simulink model "rtwdemo_PCGEvalHarness"  (Simulink 7.6)
settings: Solver=FixedStepDiscrete  StartTime=0.0  StopTime=2  FixedStep=.001  RelTol=1e-3
PostLoadFcn:
  | % Load the Data
  | RTWDemos.pcgd_TestHarnessData;
StopFcn:
  | % Run the plotting script
  | if (exist('logsout','var'))
  |     RTWDemos.pcgd_plotHarnessData(logsout);
  | end
undefined symbols (not defined in the file or in its folder): A1, A2, B0, B1, B2, sigbuilder_block
libraries: simulink x1
settings Model: Creator=The MathWorks Inc.  ExtModeAutoUpdateStatusClock=off
settings DataIOCC: SaveOutput=off  SaveTime=off
settings OptimizationCC: InitFltsAndDblsToZero=on  OptimizeModelRefInitCode=on  LifeSpan=1
settings DebuggingCC: SignalResolutionControl=TryResolveAllWithWarning  StrictBusMsg=Warning
settings ModelReferenceCC: ModelReferenceNumInstancesAllowed=Single
settings RTWCC: SystemTargetFile=ert.tlc  GenCodeOnly=on  MakeCommand="make_rtw USER_INCLUDES=\"-I$matlabroot$/toolbox\\rtw\\rtwdemos\\EmbeddedCoderOverview\\stage_4_files\""  TemplateMakefile=ert_default_tmf  Description=Real-Time Workshop Embedded Coder (no auto configuration)  ProcessScript=ert_make_rtw_hook  CustomSource=SimpleTable.c
settings RTWCC: CustomInclude=|
  | $matlabroot$\toolbox\rtw\rtwdemos\EmbeddedCoderOverview\
  | $matlabroot$\toolbox\rtw\rtwdemos\EmbeddedCoderOverview\stage_4_files
settings CodeAppCC: IgnoreCustomStorageClasses=off
settings ERTTargetCC: TargetFcnLib=ansi_tfl_tmw_new.mat  MultiwordLength=2048  GenerateSampleERTMain=on  InlinedParameterPlacement=NonHierarchical  ERTCustomFileTemplate=example_file_process.tlc  ConvertIfToSwitch=off

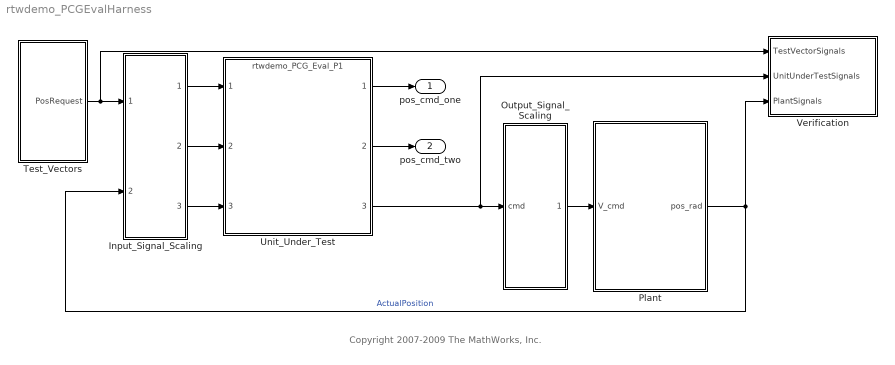
== system rtwdemo_PCGEvalHarness ==
  note: Copyright 2007-2009 The MathWorks, Inc.
  Input_Signal_Scaling : Subsystem
      mask Display:
      | disp(' ')
      | port_label('output',1,'pos_rqst');
      | port_label('output',2,'fbk_1');
      | port_label('output',3,'fbk_2');
  Output_Signal_Scaling : Subsystem
      mask Display:
      | disp(' ')
      | port_label('output',1,'pos_cmd')
  Plant : Subsystem
      mask Display: disp(' ')
  Test_Vectors : Subsystem
  Unit_Under_Test : ModelReference  ModelNameDialog=rtwdemo_PCG_Eval_P1  SimulationMode=Normal  ModelReferenceVersion=1.169  CopyOfModelName=rtwdemo_PCG_Eval_P1
  Verification : Subsystem
  pos_cmd_one : Outport
  pos_cmd_two : Outport  Port=2
  wires:
  Unit_Under_Test/3 -> Output_Signal_Scaling/1(cmd), Verification/2(UnitUnderTestSignals)
  Test_Vectors/1(PosRequest) -> Input_Signal_Scaling/1(sys_in), Verification/1(TestVectorSignals)
  Input_Signal_Scaling/1(pos_rqst) -> Unit_Under_Test/1
  Input_Signal_Scaling/2(fbk_1_out) -> Unit_Under_Test/2
  Input_Signal_Scaling/3(fbk_2_out) -> Unit_Under_Test/3
  Unit_Under_Test/1 -> pos_cmd_one/1
  Unit_Under_Test/2 -> pos_cmd_two/1
  Plant/1(pos_rad) -> Input_Signal_Scaling/2(pos_fbk), Verification/3(PlantSignals)  "ActualPosition"
  Output_Signal_Scaling/1(pos_cmd_act) -> Plant/1(V_cmd)

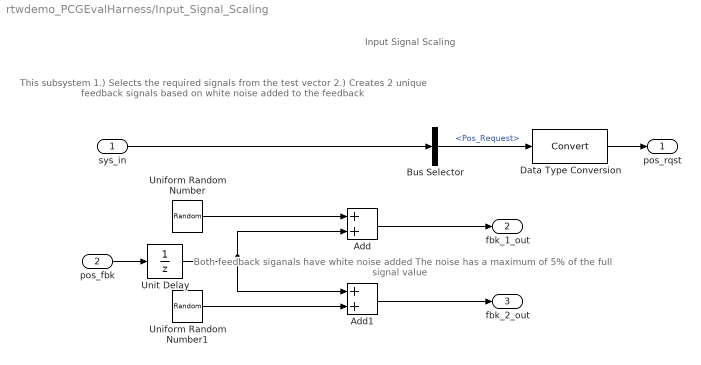
== system rtwdemo_PCGEvalHarness/Input_Signal_Scaling ==
  note: Input Signal Scaling
  note: This subsystem
      | 1.) Selects the required signals from the test vector
      | 2.) Creates 2 unique feedback signals based on white noise added to the feedback
  note: Both feedback siganals have white noise added
      | The noise has a maximum of 5% of the full signal value
  sys_in : Inport
  pos_fbk : Inport  Port=2
  Add : Sum
  Add1 : Sum
  Bus Selector : BusSelector  OutputSignals=Pos_Request
  Data Type Conversion : DataTypeConversion  SampleTime=[0.001, 0]
  Uniform Random Number : UniformRandomNumber  Minimum=-.025  Maximum=.025  SampleTime=.001
  Uniform Random Number1 : UniformRandomNumber  Minimum=-.025  Maximum=.025  Seed=10  SampleTime=.001
  Unit Delay : UnitDelay  SampleTime=-1
  pos_rqst : Outport
  fbk_1_out : Outport  Port=2
  fbk_2_out : Outport  Port=3
  wires:
  sys_in/1 -> Bus Selector/1
  Bus Selector/1 -> Data Type Conversion/1  "<Pos_Request>"
  Add/1 -> fbk_1_out/1
  Add1/1 -> fbk_2_out/1
  pos_fbk/1 -> Unit Delay/1
  Uniform Random Number/1 -> Add/1
  Uniform Random Number1/1 -> Add1/2
  Data Type Conversion/1 -> pos_rqst/1
  Unit Delay/1 -> Add/2, Add1/1

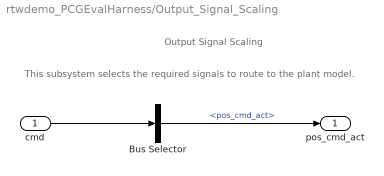
== system rtwdemo_PCGEvalHarness/Output_Signal_Scaling ==
  note: Output Signal Scaling
  note: This subsystem selects the required signals to route to the plant model.
  cmd : Inport
  Bus Selector : BusSelector  OutputSignals=pos_cmd_act
  pos_cmd_act : Outport
  wires:
  Bus Selector/1 -> pos_cmd_act/1  "<pos_cmd_act>"
  cmd/1 -> Bus Selector/1

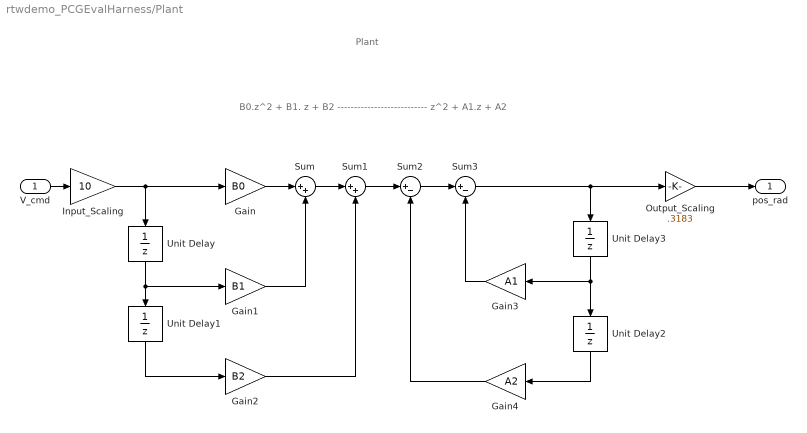
== system rtwdemo_PCGEvalHarness/Plant ==
  note: B0.z^2 + B1. z + B2
      | ---------------------------
      |    z^2 + A1.z + A2
  note: Plant
  V_cmd : Inport
  Gain : Gain  Gain=B0
  Gain1 : Gain  Gain=B1
  Gain2 : Gain  Gain=B2
  Gain3 : Gain  Gain=A1
  Gain4 : Gain  Gain=A2
  Input_Scaling : Gain  Gain=10
  Output_Scaling : Gain  Gain=.3183
  Sum : Sum  Inputs=|++
  Sum1 : Sum  Inputs=|++
  Sum2 : Sum  Inputs=|+-
  Sum3 : Sum  Inputs=|+-
  Unit Delay{,1..3} (4 alike) : UnitDelay  SampleTime=-1
  pos_rad : Outport
  wires:
  Sum2/1 -> Sum3/1
  Sum1/1 -> Sum2/1
  Gain4/1 -> Sum2/2
  Unit Delay2/1 -> Gain4/1
  Gain3/1 -> Sum3/2
  Unit Delay3/1 -> Unit Delay2/1, Gain3/1
  Sum3/1 -> Unit Delay3/1, Output_Scaling/1
  Gain2/1 -> Sum1/2
  Sum/1 -> Sum1/1
  Gain1/1 -> Sum/2
  Gain/1 -> Sum/1
  Unit Delay1/1 -> Gain2/1
  Unit Delay/1 -> Unit Delay1/1, Gain1/1
  V_cmd/1 -> Input_Scaling/1
  Output_Scaling/1 -> pos_rad/1
  Input_Scaling/1 -> Unit Delay/1, Gain/1

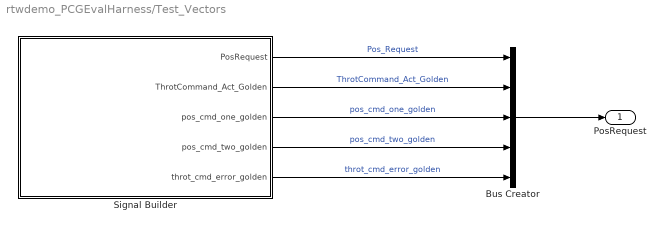
== system rtwdemo_PCGEvalHarness/Test_Vectors ==
  Bus Creator : BusCreator  Inputs=5
  Signal Builder : Subsystem  Tag=STV Subsys  LoadFcn=sigbuilder_block('load');  StartFcn=sigbuilder_block('start');  StopFcn=sigbuilder_block('stop');  ClipboardFcn=sigbuilder_block('clipboard');  mask(Sigbuilder block){}
      mask help: Sigbuilder GUI
      mask init:
      | if ~strcmp(get_param(bdroot(gcbh),'SimulationStatus'),'stopped') tuvar = sigbuilder_block('maskInit'); end
      settings: CopyFcn=sigbuilder_block('copy');  DeleteFcn=sigbuilder_block('delete');  ModelCloseFcn=sigbuilder_block('modelClose');  PreSaveFcn=sigbuilder_block('preSave');  NameChangeFcn=sigbuilder_block('namechange');  OpenFcn=sigbuilder_block('open',[0 25.5 1248 819 ]);  CloseFcn=sigbuilder_block('close');
      mask Display: plot(0,0,100,100,[10,10,40,40,10],[80,20,20,80,80],[40,10],[50,50], [40,27,10],[65,72,56],[40,25,25,10],[28,28,43,43]);
  PosRequest : Outport
  wires:
  Bus Creator/1 -> PosRequest/1
  Signal Builder/1(PosRequest) -> Bus Creator/1  "Pos_Request"
  Signal Builder/2(ThrotCommand_Act_Golden) -> Bus Creator/2  "ThrotCommand_Act_Golden"
  Signal Builder/3(pos_cmd_one_golden) -> Bus Creator/3  "pos_cmd_one_golden"
  Signal Builder/4(pos_cmd_two_golden) -> Bus Creator/4  "pos_cmd_two_golden"
  Signal Builder/5(throt_cmd_error_golden) -> Bus Creator/5  "throt_cmd_error_golden"

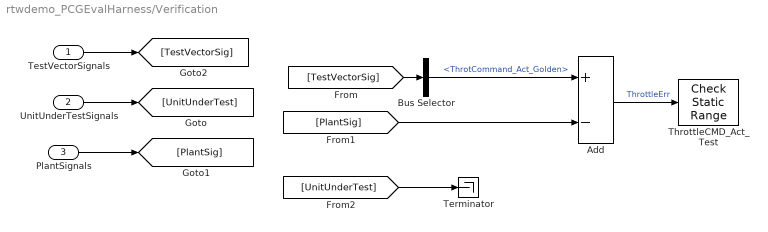
== system rtwdemo_PCGEvalHarness/Verification ==
  TestVectorSignals : Inport
  UnitUnderTestSignals : Inport  Port=2
  PlantSignals : Inport  Port=3
  Add : Sum  Inputs=+-
  Bus Selector : BusSelector  OutputSignals=ThrotCommand_Act_Golden
  Terminator : Terminator
  ThrottleCMD_Act_Test : simulink/Model Verification/Check  Static Range  Description=-.05 <= u <= .05  SystemSampleTime=-1  max=.05  max_included=on  min=-.05  min_included=on  enabled=on  stopWhenAssertionFail=off  export=off  icon=graphic
  wires:
  UnitUnderTestSignals/1 -> [UnitUnderTest]
  PlantSignals/1 -> [PlantSig]
  TestVectorSignals/1 -> [TestVectorSig]
  [TestVectorSig] -> Bus Selector/1
  Bus Selector/1 -> Add/1  "<ThrotCommand_Act_Golden>"
  [PlantSig] -> Add/2
  Add/1 -> ThrottleCMD_Act_Test/1  "ThrottleErr"
  [UnitUnderTest] -> Terminator/1

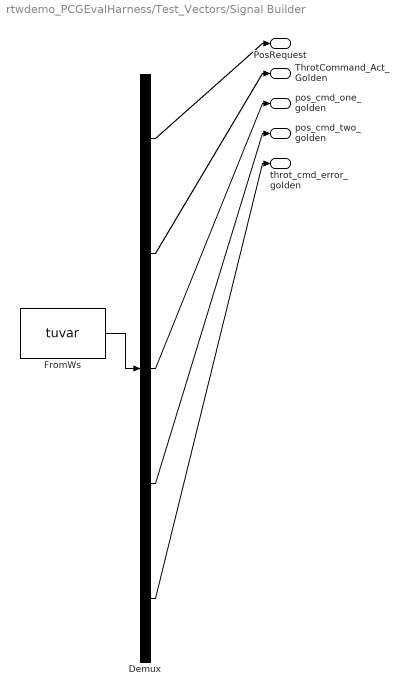
== system rtwdemo_PCGEvalHarness/Test_Vectors/Signal Builder ==
  Demux : Demux  Tag=STV Demux  Outputs=5
  FromWs : FromWorkspace  Tag=STV FromWs  VariableName=tuvar  SampleTime=0  SigBuilderData=DataTag0  VnvData=DataTag1
      SigBuilderData=|
      | common.afterFinalStr = 'Extrapolate'
      | common.sampleTime = 0
      | dataSet.timeRange = [0 2]
      | dataSet.name = 'Group 1'
      | sbobj.Groups.Name = 'Group 1'
      | sbobj.Groups.Signals(1).Name = 'PosRequest'
      | sbobj.Groups.Signals(1).XData = [0 0.19 0.19 0.605 0.605 1.26 1.405 2]
      | sbobj.Groups.Signals(1).YData = [0 0 1 1 0.5 0.55 -0.2 0.55]
      | sbobj.Groups.Signals(2).Name = 'ThrotCommand_Act_Golden'
      | sbobj.Groups.Signals(2).XData = [0 0.001 0.002 0.003 0.004 0.005 0.006 0.007 0.008 0.009 0.01 0.011 ... (2001 elements, 1x2001)]
      | sbobj.Groups.Signals(2).YData = [0 1.39704476074e-07 4.11080420847e-07 6.66852248796e-07 9.07917196637e-07 1.13512090998e-06 1.3492604098e-06 1.55108688839e-06 1.60197461553e-06 1.51060256944e-06 1.42448441599e-06 1.34331805638e-06 ... (2001 elements, 1x2001)]
      | sbobj.Groups.Signals(3).Name = 'pos_cmd_one_golden'
      | sbobj.Groups.Signals(3).XData = [0 0.001 0.002 0.003 0.004 0.005 0.006 0.007 0.008 0.009 0.01 0.011 ... (2001 elements, 1x2001)]
      | sbobj.Groups.Signals(3).YData = [4.38908187476e-05 0.000220800396297 0 0 -0.000196616963999 0 0 -8.35534330088e-05 0.000238023449227 0.00021210757514 0 0 ... (2001 elements, 1x2001)]
      | sbobj.Groups.Signals(4).Name = 'pos_cmd_two_golden'
      | sbobj.Groups.Signals(4).XData = [0 0.001 0.002 0.003 0.004 0.005 0.006 0.007 0.008 0.009 0.01 0.011 ... (2001 elements, 1x2001)]
      | sbobj.Groups.Signals(4).YData = [0.000122162776717 0 0 -0.000217425331739 0 0.000163100882168 9.20021833969e-05 -4.37743414776e-05 0 0 -0.000179958926357 -5.6098985519e-06 ... (2001 elements, 1x2001)]
      | sbobj.Groups.Signals(5).Name = 'throt_cmd_error_golden'
      | sbobj.Groups.Signals(5).XData = [0 2]
      | sbobj.Groups.Signals(5).YData = [0 0]
      | sbobj.Groups.TimeRange = [0 2]
  PosRequest : Outport  Tag=STV Outport
  ThrotCommand_Act_Golden : Outport  Tag=STV Outport  Port=2
  pos_cmd_one_golden : Outport  Tag=STV Outport  Port=3
  pos_cmd_two_golden : Outport  Tag=STV Outport  Port=4
  throt_cmd_error_golden : Outport  Tag=STV Outport  Port=5
  wires:
  FromWs/1 -> Demux/1
  Demux/1 -> PosRequest/1
  Demux/2 -> ThrotCommand_Act_Golden/1
  Demux/3 -> pos_cmd_one_golden/1
  Demux/4 -> pos_cmd_two_golden/1
  Demux/5 -> throt_cmd_error_golden/1
